simulink model "Edge_detector_HIL"  (Simulink 7.0)
settings: Solver=FixedStepDiscrete  SolverMode=SingleTasking  StartTime=0.0  StopTime=307201.0  RelTol=1e-3
InitFcn:
  | ed_in_script
  | %% DSPBuilder Start
  | alt_dspbuilder_update_model(bdroot)
  | %% DSPBuilder End
StopFcn:
  | ed_out_script
libraries: allblocks_alteradspbuilder2 x8
settings Model: Creator=lkong  LastModifiedBy=lkong
settings DataIOCC: SignalLoggingName=sigsOut
settings OptimizationCC: InlineInvariantSignals=on
settings DebuggingCC: SaveWithParameterizedLinksMsg=none  SignalResolutionControl=TryResolveAllWithWarning  SolverPrmCheckMsg=none  MultiTaskDSMMsg=warning  MultiTaskCondExecSysMsg=none  StrictBusMsg=None
settings HardwareCC: TargetUnknown=on
settings RTWCC: IncludeERTFirstTime=on
settings GRTTargetCC: TargetFcnLib=ansi_tfl_tmw.mat

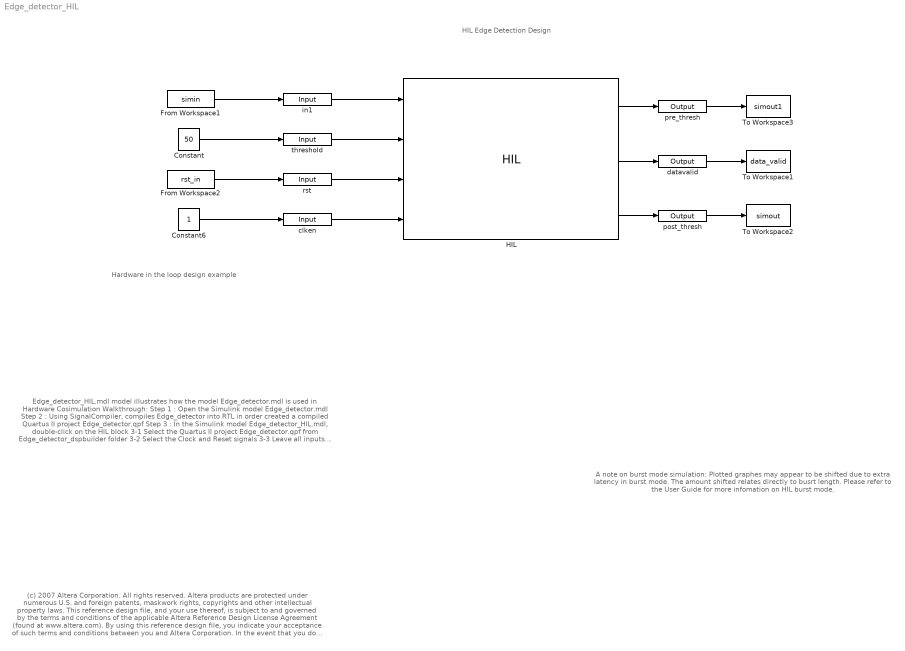
== system Edge_detector_HIL ==
  note: HIL Edge Detection Design
  note: (c) 2007 Altera Corporation. All rights reserved.  Altera products are protected under numerous U.S. and foreign patents, maskwork rights, copyrights and other intellectual property laws.
      | This reference design file, and your use thereof, is subject to and governed by the terms and conditions of the applicable Altera Reference Design License Agreement (found at www.altera.com).
      | By using this reference design file, you indicate your acceptance of such terms and conditions between you and Altera Corporation.
      | In the event that you do not agree with such terms and conditions, you may not use the reference design file and please promptly destroy any copies you have made.
      | This reference design file being provided on an "as-is" basis and as an accommodation and therefore all warranties, representations or guarantees of any kind (whether express, implied or statutory)
      | including, without limitation, warranties of merchantability, non-infringement, or fitness for a particular purpose, are specifically disclaimed.
      | By making this reference design file available, Altera expressly does not recommend, suggest or require that this reference design file be used in combination with any other product not provided by Altera
  note: Hardware in the loop design example
  note: Edge_detector_HIL.mdl model illustrates how the model Edge_detector.mdl is used in Hardware Cosimulation
      |
      | Walkthrough:
      | Step 1 : Open the Simulink model Edge_detector.mdl
      | Step 2 : Using SignalCompiler, compiles Edge_detector into RTL in order created a compiled Quartus II project Edge_detector.qpf
      | Step 3 : In the Simulink model Edge_detector_HIL.mdl, double-click on the HIL block
      |               3-1 Select the Quartus II project Edge_detector.qpf from Edge_detector_dspbuilder folder
      |               3-2 Select the Clock and Reset signals
      |               3-3 Leave all inputs and outputs as unsigned
      |               3-4 Select the reset active level
      |               3-5 Click on Goto page 2/2
      |               3-6 Enter the FPGA device value
      |               3-7 Compile with Quartus II
      |               3-8 Scan JTAG and Select the JTAG cable
      |               3-9 Program the FPGA on board
      |               3-10 Close the HIL dialog box
      |
      | Step 4 : Simulate in Simulink
  note: A note on burst mode simulation:
      |
      |     Plotted graphes may appear to be shifted
      | due to extra latency in burst mode. The amount
      | shifted relates directly to busrt length.
      |
      |     Please refer to the User Guide for more
      | infomation on HIL burst mode.
  Constant : Constant  Value=50  OutDataType=sfix(16)  OutScaling=2^0
  Constant6 : Constant  OutDataType=sfix(16)  OutScaling=2^0
  From Workspace1 : FromWorkspace  VariableName=simin  SampleTime=1
  From Workspace2 : FromWorkspace  VariableName=rst_in  SampleTime=1
  HIL : allblocks_alteradspbuilder2/HIL  entityName=Edge_detector_HIL/HIL  inNames=in1 threshold rst clken  inBwls="8  8  1  1  1  1"  inBwrs="0  0  0  0  0  0"  inTypes=u u u u  inDelayed="1  1  1  1"  outNames=pre_thresh datavalid post_thresh  outBwls="8  1  8"  outBwrs="0  0  0"  outTypes=u u u  resetNames=aclr  InputCount=6  InputNames=in1 Clock threshold rst clken aclr  InputWidth="8  1  8  1  1  1"  InputRepresentation="0  0  0  0  0  0"  InputExport="0  2  0  0  0  3"  InputFPP="0  0  0  0  0  0"  OutputCount=3  OutputNames=pre_thresh datavalid post_thresh  OutputWidth="8  1  8"  OutputRepresentation="0  0  0"  OutputExport="0  0  0"  OutputFPP="0  0  0"  JtagCable=3  JtagDevice=1  BurstMode=on  BurstLength=1024  FrameMode=off  SOP=1  OutValid=1  QuartusProject=D:\workspace\Documentation\DesignExamples\Tutorials\HIL\EdgeDetection\Edge_detector_dspbuilder\Edge_detector.qpf  HilNewConfig=off  ClockPinLocation=K17  ClockPinSource=0  HilDeviceOnBoard=EP2S60F1020C5  DR_length=24  dspbuilder_reset=on  SLD_NODE_INFO=10036336  AssertSclrBeforeSimulation=1  SampleTime=-1  dspb_ver=5.1  ResetLevel=Active_High  JtagCableName=USB-Blaster [USB-0]  JtagDeviceName=@1: EP2S60 (0x120930DD)  ClockNames=Clock
  To Workspace1 : ToWorkspace  VariableName=data_valid  SaveFormat=Array
  To Workspace2 : ToWorkspace  VariableName=simout  SaveFormat=Array
  To Workspace3 : ToWorkspace  VariableName=simout1  SaveFormat=Array
  clken : allblocks_alteradspbuilder2/Input  iofile=d:\p4DspbStd81\P4ws\dsp_builder2\Documentation\DesignExamples\Tutorials\HIL\EdgeDetection\tb_Edge_detector_HIL\Edge%5Fdetector%5FHIL_clken.salt  BusType=Single Bit  bwl=1  bwr=0  SpecifyClock=off  PORTTYPE=Input  externalType=Inferred  allowFloatingPointOverride=on  logOutputs=off
  datavalid : allblocks_alteradspbuilder2/Output  iofile=d:\p4DspbStd81\P4ws\dsp_builder2\Documentation\DesignExamples\Tutorials\HIL\EdgeDetection\tb_Edge_detector_HIL\Edge%5Fdetector%5FHIL_datavalid.capture  BusType=Single Bit  bwl=1  bwr=0  externalType=Inferred  PORTTYPE=Output  allowFloatingPointOverride=on  logOutputs=off
  in1 : allblocks_alteradspbuilder2/Input  iofile=d:\p4DspbStd81\P4ws\dsp_builder2\Documentation\DesignExamples\Tutorials\HIL\EdgeDetection\tb_Edge_detector_HIL\Edge%5Fdetector%5FHIL_in1.salt  BusType=Unsigned Integer  bwl=8  bwr=0  SpecifyClock=off  PORTTYPE=Input  externalType=Inferred  allowFloatingPointOverride=on  logOutputs=off
  post_thresh : allblocks_alteradspbuilder2/Output  iofile=d:\p4DspbStd81\P4ws\dsp_builder2\Documentation\DesignExamples\Tutorials\HIL\EdgeDetection\tb_Edge_detector_HIL\Edge%5Fdetector%5FHIL_post%5Fthresh.capture  BusType=Unsigned Integer  bwl=8  bwr=0  externalType=Inferred  PORTTYPE=Output  allowFloatingPointOverride=on  logOutputs=off
  pre_thresh : allblocks_alteradspbuilder2/Output  iofile=d:\p4DspbStd81\P4ws\dsp_builder2\Documentation\DesignExamples\Tutorials\HIL\EdgeDetection\tb_Edge_detector_HIL\Edge%5Fdetector%5FHIL_pre%5Fthresh.capture  BusType=Unsigned Integer  bwl=8  bwr=0  externalType=Inferred  PORTTYPE=Output  allowFloatingPointOverride=on  logOutputs=off
  rst : allblocks_alteradspbuilder2/Input  iofile=d:\p4DspbStd81\P4ws\dsp_builder2\Documentation\DesignExamples\Tutorials\HIL\EdgeDetection\tb_Edge_detector_HIL\Edge%5Fdetector%5FHIL_rst.salt  BusType=Single Bit  bwl=1  bwr=0  SpecifyClock=off  PORTTYPE=Input  externalType=Inferred  allowFloatingPointOverride=on  logOutputs=off
  threshold : allblocks_alteradspbuilder2/Input  iofile=d:\p4DspbStd81\P4ws\dsp_builder2\Documentation\DesignExamples\Tutorials\HIL\EdgeDetection\tb_Edge_detector_HIL\Edge%5Fdetector%5FHIL_threshold.salt  BusType=Unsigned Integer  bwl=8  bwr=0  SpecifyClock=off  PORTTYPE=Input  externalType=Inferred  allowFloatingPointOverride=on  logOutputs=off
  wires:
  Constant6/1 -> clken/1
  Constant/1 -> threshold/1
  From Workspace2/1 -> rst/1
  From Workspace1/1 -> in1/1
  datavalid/1 -> To Workspace1/1
  pre_thresh/1 -> To Workspace3/1
  post_thresh/1 -> To Workspace2/1
  clken/1 -> HIL/4
  rst/1 -> HIL/3
  threshold/1 -> HIL/2
  in1/1 -> HIL/1
  HIL/3 -> post_thresh/1
  HIL/1 -> pre_thresh/1
  HIL/2 -> datavalid/1
